simulink model "ref_submodel3"  (R2022b)
settings: Solver=FixedStepDiscrete  StartTime=0.0  StopTime=inf  RelTol=1e-3  EnableMultiTasking=on
values from neighbouring files (symbols this model uses):
  ts = 1e-4    (= 0.0001)    [main_test.m]
libraries: speedgoatlib_IO104 x2
settings Model: Creator=dmankov  LastModifiedBy=padlewsk
settings SolverCC: ConcurrentTasks=on  AlgebraicLoopSolver=TrustRegion  PositivePriorityOrder=on  AutoInsertRateTranBlk=on  InsertRTBMode=Never (minimum delay)
settings DataIOCC: SaveFormat=StructureWithTime
settings OptimizationCC: BlockReduction=off  OptimizeBlockIOStorage=off  BufferReuse=off  ReuseModelBlockBuffer=on  GlobalBufferReuse=off  ExpressionFolding=off  LocalBlockOutputs=off  OptimizeDataStoreBuffers=off  BusAssignmentInplaceUpdate=off
settings DebuggingCC: TasksWithSamePriorityMsg=none  UnconnectedInputMsg=warning  UnconnectedOutputMsg=warning  UnconnectedLineMsg=warning  ArithmeticOperatorsInVariantConditions=warning
settings HardwareCC: ProdBitPerLong=64  ProdLongLongMode=on  ProdHWDeviceType=Intel->x86-64 (Linux 64)
settings ModelReferenceCC: EnableRefExpFcnMdlSchedulingChecks=on  ModelReferenceNumInstancesAllowed=Single
settings SFSimCC: CustomCodeUndefinedFunction=UseInterfaceOnly
settings RTWCC: Description=Simulink Real-Time  SystemTargetFile=slrealtime.tlc  TemplateMakefile=slrealtime_default_tmf  Toolchain=Simulink Real-Time Toolchain  BuildConfiguration=Faster Runs  CodeExecutionProfiling=on  TargetLang=C++  DLArmComputeVersion=19.05
settings SimulinkRealTimeTargetCC: UseGCCFastMath=on

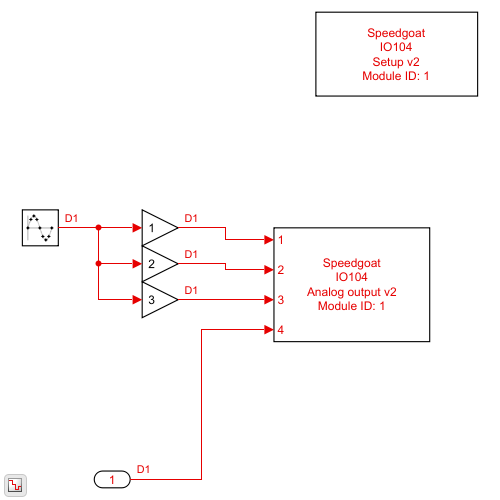
[thumbnail: Simulink's stored preview of the top-level diagram]
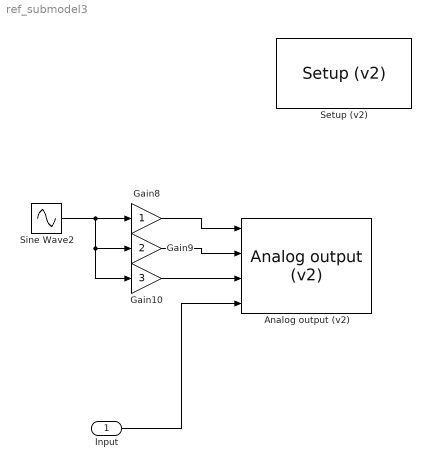
== system ref_submodel3 ==
  Input : Inport
  "Analog output (v2) " : speedgoatlib_IO104/Analog output (v2)   parModuleId=1  parTs=-1  parPciSlot=-1  parDaSimultaneous=on  parDaChannels=[1,2,3,4]  parDaChannelsSorted=[1,2,3,4]  parDaInitValue=[0,0,0,0]  parDaReset=[1,1,1,1]  parDaRange=+-10V  parDaFrameSize=1  parDaUseTrigger=on  parDaClockInitiator=Initiator  parDaSampleTime=4.000000000e-04  parTriggerInitiator=Target  parTriggerRate=1.000000000e-03  parAdBlockPresent=0
      settings: SourceProductName=Simulink Real-Time: Speedgoat I/O Blockset
  Gain10 : Gain  Gain=3
  Gain8 : Gain
  Gain9 : Gain  Gain=2
  "Setup (v2) " : speedgoatlib_IO104/Setup (v2)   parPciSlot=-1  parModuleId=1  parTriggerInitiator=Target  parTriggerRate=1e-3  parCalibrate=off  parAdChannels=[1:8]  parAdRange1=+-10V  parAdRange2=+-10V  parAdCoupling=Differential  parAdUseTrigger=on  parAdFrameSize=1  parAdClockInitiator=Initiator  parAdSampleTime=400e-6  parDaSimultaneous=on  parDaChannels=[1:4]  parDaChannelsSorted=[1,2,3,4]  parDaInitValue=[0]  parDaReset=[1]  parDaRange=+-10V  parDaUseTrigger=on  parDaFrameSize=1  parDaClockInitiator=Initiator  parDaSampleTime=400e-6  parDioByte0Dir=Outputs  parDioByte1Dir=Inputs  parDoChannels=[1:4]  parDoInitValues=[0]  parDoReset=[1]  parDiChannels=[13:16]
      settings: SourceProductName=Simulink Real-Time: Speedgoat I/O Blockset
  Sine Wave2 : Sin  SineType=Sample based  Samples=50  SampleTime=ts
  wires:
  Input/1 -> "Analog output (v2) "/4
  Sine Wave2/1 -> Gain8/1, Gain10/1, Gain9/1
  Gain8/1 -> "Analog output (v2) "/1
  Gain9/1 -> "Analog output (v2) "/2
  Gain10/1 -> "Analog output (v2) "/3
